simulink model "on_off_example"  (R2017a)
settings: Solver=FixedStepDiscrete  StartTime=1  StopTime=500  FixedStep=1  RelTol=1e-3
settings Model: Creator=zhiangz  LastModifiedBy=zhiangz

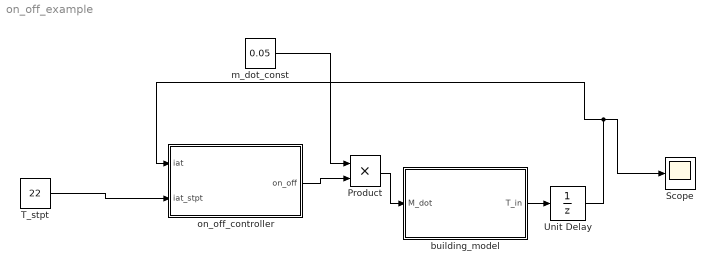
== system on_off_example ==
  Product : Product
  Scope : Scope
  T_stpt : Constant  Value=22
  Unit Delay : UnitDelay  SampleTime=-1
  building_model : Subsystem
  m_dot_const : Constant  Value=0.05
  on_off_controller : Subsystem
  wires:
  building_model/1(T_in) -> Unit Delay/1
  T_stpt/1 -> on_off_controller/2(iat_stpt)
  Product/1 -> building_model/1(M_dot)
  m_dot_const/1 -> Product/1
  on_off_controller/1(on_off) -> Product/2
  Unit Delay/1 -> on_off_controller/1(iat), Scope/1

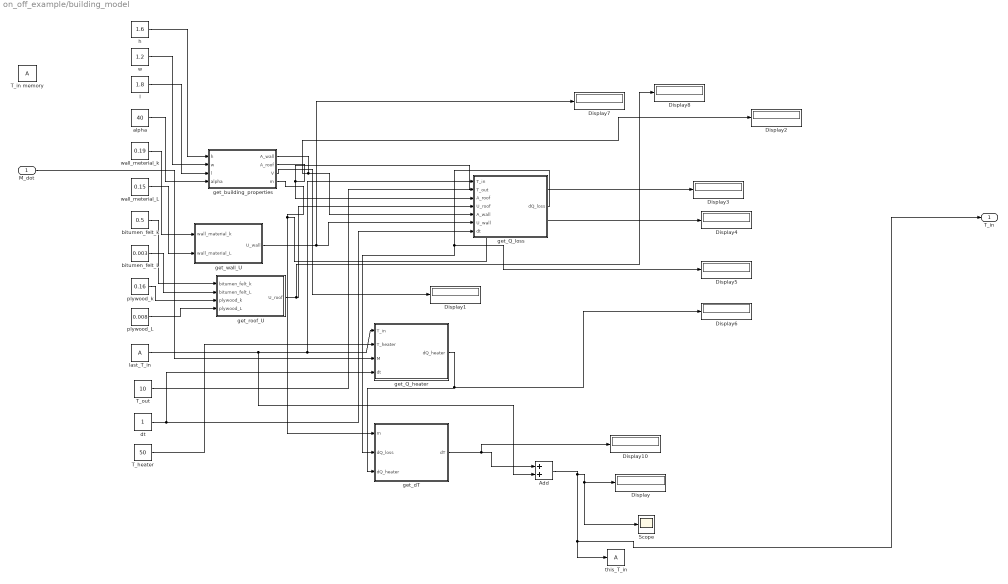
== system on_off_example/building_model ==
  M_dot : Inport
  Add : Sum
  Display{,1..8,10} (10 alike) : Display
  Scope : Scope
  T_heater : Constant  Value=50
  T_in memory : DataStoreMemory  ReadBeforeWriteMsg=warning  WriteAfterWriteMsg=warning  WriteAfterReadMsg=warning  InitialValue=10  ShowAdditionalParam=off
  T_out : Constant  Value=10
  alpha : Constant  Value=40
  bitumen_felt_L : Constant  Value=0.003
  bitumen_felt_k : Constant  Value=0.5
  dt : Constant
  get_Q_heater : Subsystem
  get_Q_loss : Subsystem
  get_building_properties : Subsystem
  get_dT : Subsystem
  get_roof_U : Subsystem
  get_wall_U : Subsystem
  h : Constant  Value=1.6
  l : Constant  Value=1.8
  last_T_in : DataStoreRead
  plywood_L : Constant  Value=0.008
  plywood_k : Constant  Value=0.16
  this_T_in : DataStoreWrite
  w : Constant  Value=1.2
  wall_meterial_L : Constant  Value=0.15
  wall_meterial_k : Constant  Value=0.19
  T_in : Outport
  wires:
  last_T_in/1 -> Add/2, get_Q_heater/1(T_in), get_Q_loss/1(T_in)
  T_heater/1 -> get_Q_heater/2(T_heater)
  get_building_properties/4(m) -> Display4/1, get_dT/1(m)
  get_roof_U/1(U_roof) -> Display8/1, get_Q_loss/4(U_roof)
  bitumen_felt_k/1 -> get_roof_U/1(bitumen_felt_k)
  get_building_properties/3(V) -> Display1/1
  w/1 -> get_building_properties/2(w)
  get_building_properties/2(A_roof) -> Display3/1, get_Q_loss/3(A_roof)
  dt/1 -> get_Q_heater/4(dt), get_Q_loss/7(dt)
  M_dot/1 -> get_Q_heater/3(M)
  get_wall_U/1(U_wall) -> Display7/1, get_Q_loss/6(U_wall)
  Add/1 -> Scope/1, Display/1, T_in/1, this_T_in/1
  get_building_properties/1(A_wall) -> Display2/1, get_Q_loss/5(A_wall)
  h/1 -> get_building_properties/1(h)
  wall_meterial_L/1 -> get_wall_U/2(wall_material_L)
  wall_meterial_k/1 -> get_wall_U/1(wall_material_k)
  bitumen_felt_L/1 -> get_roof_U/2(bitumen_felt_L)
  T_out/1 -> get_Q_loss/2(T_out)
  l/1 -> get_building_properties/3(l)
  get_Q_heater/1(dQ_heater) -> Display6/1, get_dT/3(dQ_heater)
  plywood_L/1 -> get_roof_U/4(plywood_L)
  get_Q_loss/1(dQ_loss) -> Display5/1, get_dT/2(dQ_loss)
  plywood_k/1 -> get_roof_U/3(plywood_k)
  alpha/1 -> get_building_properties/4(alpha)
  get_dT/1(dT) -> Display10/1, Add/1

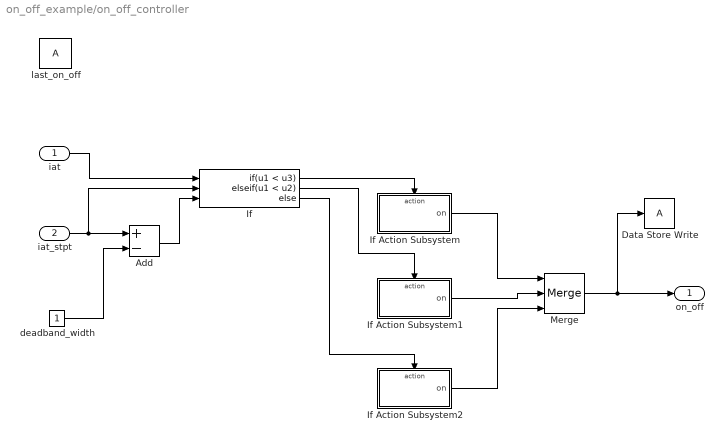
== system on_off_example/on_off_controller ==
  iat : Inport
  iat_stpt : Inport  Port=2
  Add : Sum  Inputs=+-
  Data Store Write : DataStoreWrite
  If : If  NumInputs=3  IfExpression=u1 < u3  ElseIfExpressions=u1 < u2
  If Action Subsystem : Subsystem  TreatAsAtomicUnit=on
  If Action Subsystem1 : Subsystem  TreatAsAtomicUnit=on
  If Action Subsystem2 : Subsystem  TreatAsAtomicUnit=on
  Merge : Merge  Inputs=3
  deadband_width : Constant
  last_on_off : DataStoreMemory  ReadBeforeWriteMsg=warning  WriteAfterWriteMsg=warning  WriteAfterReadMsg=warning  ShowAdditionalParam=off
  on_off : Outport
  wires:
  iat/1 -> If/1
  iat_stpt/1 -> Add/1, If/2
  deadband_width/1 -> Add/2
  Add/1 -> If/3
  If/1 -> If Action Subsystem/Action
  If/2 -> If Action Subsystem1/Action
  If/3 -> If Action Subsystem2/Action
  If Action Subsystem/1(on) -> Merge/1
  If Action Subsystem1/1(on) -> Merge/2
  If Action Subsystem2/1(on) -> Merge/3
  Merge/1 -> Data Store Write/1, on_off/1

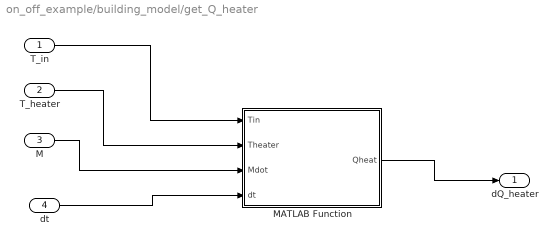
== system on_off_example/building_model/get_Q_heater ==
  T_in : Inport
  T_heater : Inport  Port=2
  M : Inport  Port=3
  dt : Inport  Port=4
  MATLAB Function : MATLAB Function  TreatAsAtomicUnit=on
  dQ_heater : Outport
  wires:
  T_in/1 -> MATLAB Function/1(Tin)
  T_heater/1 -> MATLAB Function/2(Theater)
  M/1 -> MATLAB Function/3(Mdot)
  dt/1 -> MATLAB Function/4(dt)
  MATLAB Function/1(Qheat) -> dQ_heater/1

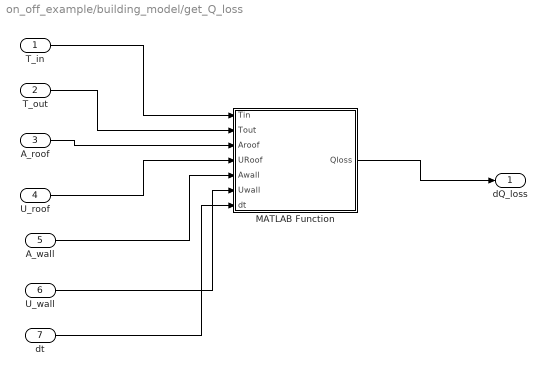
== system on_off_example/building_model/get_Q_loss ==
  T_in : Inport
  T_out : Inport  Port=2
  A_roof : Inport  Port=3
  U_roof : Inport  Port=4
  A_wall : Inport  Port=5
  U_wall : Inport  Port=6
  dt : Inport  Port=7
  MATLAB Function : MATLAB Function  TreatAsAtomicUnit=on
  dQ_loss : Outport
  wires:
  T_in/1 -> MATLAB Function/1(Tin)
  T_out/1 -> MATLAB Function/2(Tout)
  A_roof/1 -> MATLAB Function/3(Aroof)
  U_roof/1 -> MATLAB Function/4(URoof)
  A_wall/1 -> MATLAB Function/5(Awall)
  U_wall/1 -> MATLAB Function/6(Uwall)
  dt/1 -> MATLAB Function/7(dt)
  MATLAB Function/1(Qloss) -> dQ_loss/1

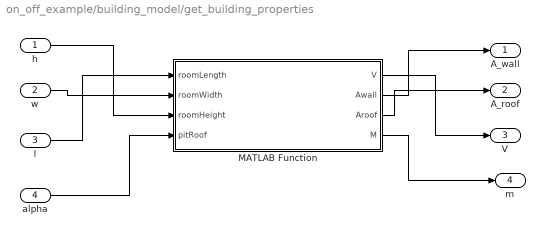
== system on_off_example/building_model/get_building_properties ==
  h : Inport
  w : Inport  Port=2
  l : Inport  Port=3
  alpha : Inport  Port=4
  MATLAB Function : MATLAB Function  TreatAsAtomicUnit=on
  A_wall : Outport
  A_roof : Outport  Port=2
  V : Outport  Port=3
  m : Outport  Port=4
  wires:
  h/1 -> MATLAB Function/3(roomHeight)
  w/1 -> MATLAB Function/2(roomWidth)
  l/1 -> MATLAB Function/1(roomLength)
  alpha/1 -> MATLAB Function/4(pitRoof)
  MATLAB Function/1(V) -> V/1
  MATLAB Function/2(Awall) -> A_wall/1
  MATLAB Function/3(Aroof) -> A_roof/1
  MATLAB Function/4(M) -> m/1

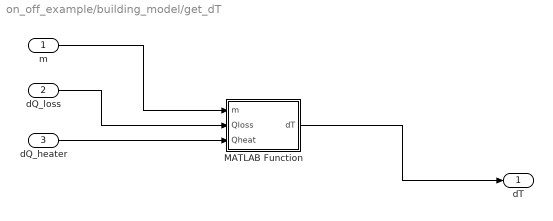
== system on_off_example/building_model/get_dT ==
  m : Inport
  dQ_loss : Inport  Port=2
  dQ_heater : Inport  Port=3
  MATLAB Function : MATLAB Function  TreatAsAtomicUnit=on
  dT : Outport
  wires:
  m/1 -> MATLAB Function/1(m)
  dQ_loss/1 -> MATLAB Function/2(Qloss)
  dQ_heater/1 -> MATLAB Function/3(Qheat)
  MATLAB Function/1(dT) -> dT/1

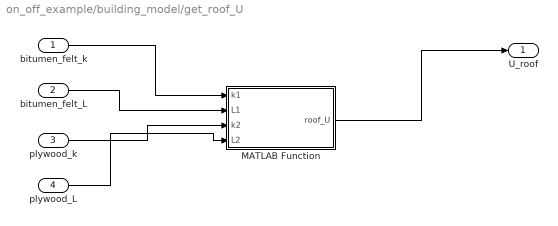
== system on_off_example/building_model/get_roof_U ==
  bitumen_felt_k : Inport
  bitumen_felt_L : Inport  Port=2
  plywood_k : Inport  Port=3
  plywood_L : Inport  Port=4
  MATLAB Function : MATLAB Function  TreatAsAtomicUnit=on
  U_roof : Outport
  wires:
  bitumen_felt_k/1 -> MATLAB Function/1(k1)
  bitumen_felt_L/1 -> MATLAB Function/2(L1)
  plywood_k/1 -> MATLAB Function/3(k2)
  plywood_L/1 -> MATLAB Function/4(L2)
  MATLAB Function/1(roof_U) -> U_roof/1

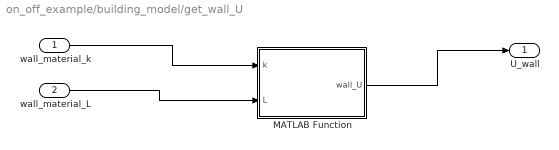
== system on_off_example/building_model/get_wall_U ==
  wall_material_k : Inport
  wall_material_L : Inport  Port=2
  MATLAB Function : MATLAB Function  TreatAsAtomicUnit=on
  U_wall : Outport
  wires:
  wall_material_k/1 -> MATLAB Function/1(k)
  wall_material_L/1 -> MATLAB Function/2(L)
  MATLAB Function/1(wall_U) -> U_wall/1

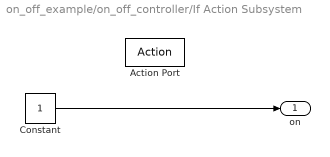
== system on_off_example/on_off_controller/If Action Subsystem ==
  Action Port : ActionPort  ActionType=then
  Constant : Constant
  on : Outport
  wires:
  Constant/1 -> on/1

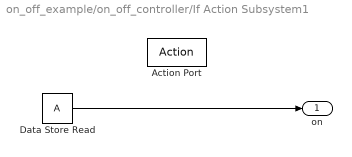
== system on_off_example/on_off_controller/If Action Subsystem1 ==
  Action Port : ActionPort  ActionType=elseif
  Data Store Read : DataStoreRead
  on : Outport
  wires:
  Data Store Read/1 -> on/1

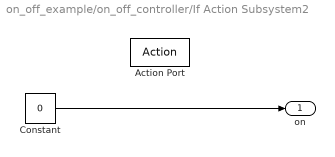
== system on_off_example/on_off_controller/If Action Subsystem2 ==
  Action Port : ActionPort  ActionType=else
  Constant : Constant  Value=0
  on : Outport
  wires:
  Constant/1 -> on/1

== matlab function on_off_example/building_model/get_wall_U/MATLAB Function ==
  data: k input; wall_U output; L input
function wall_U = getWallU(k, L)
wall_U = k/L;

== matlab function on_off_example/building_model/get_building_properties/MATLAB Function ==
  data: roomLength input; V output; roomWidth input; roomHeight input; pitRoof input; Awall output; Aroof output; M output
function [V, Awall,Aroof, M] = buildingProperties(roomLength,roomWidth,roomHeight,pitRoof)
% Your Name

densAir = 1.2250;

Awall = 2*roomLength*roomHeight;
Awall = Awall+ 2*roomWidth*roomHeight;
Awall = Awall + 0.5*tand(pitRoof)*roomWidth^2;

Aroof = (1/cosd(pitRoof))*roomWidth*roomLength;

V = roomLength * roomWidth * roomHeight;
V = V + (roomLength * roomWidth * tand(pitRoof)*roomWidth/2)/2;

M = V*densAir;
end

== matlab function on_off_example/building_model/get_roof_U/MATLAB Function ==
  data: k1 input; roof_U output; L1 input; k2 input; L2 input
function roof_U = getRoofU(k1, L1, k2, L2)
Rroof = L1/k1 + L2/k2;
roof_U = 1/Rroof;

== matlab function on_off_example/building_model/get_Q_loss/MATLAB Function ==
  data: Tin input; Qloss output; Tout input; Aroof input; URoof input; Awall input; Uwall input; dt input
function Qloss  = getQloss(Tin,Tout,Aroof,URoof,Awall,Uwall,dt)
% Your Name

    dT = Tin - Tout;
    Qloss = dT*Aroof*URoof*dt + dT*Awall*Uwall*dt;    
    
end

== matlab function on_off_example/building_model/get_Q_heater/MATLAB Function ==
  data: Tin input; Qheat output; Theater input; Mdot input; dt input
function Qheat  = getQheater(Tin,Theater,Mdot,dt)
% Your Name

    c = 1005.4;    
    dT = Theater - Tin;
    Qheat =  dT*Mdot*c*dt;
    
end

== matlab function on_off_example/building_model/get_dT/MATLAB Function ==
  data: m input; dT output; Qloss input; Qheat input
function dT  = getdT(m,Qloss,Qheat)
% Your Name

    c = 1005.4;  
    dT = (1/(m*c))*(Qheat - Qloss);
    
end
